simulink model "path_following_control"  (R2021a)
settings: Solver=VariableStepAuto  StartTime=0.0  StopTime=sim_time  RelTol=1e-3
values from neighbouring files (symbols this model uses):
  amax_ego = 3    [Combined_Control_Model.m]
  amin_ego = -3    [Combined_Control_Model.m]
  Cf = 155494.663    [Combined_Control_Model.m]
  Cr = 1554494.663    [Combined_Control_Model.m]
  D_default = 10    [Combined_Control_Model.m]
  Iz = 1436.24    [Combined_Control_Model.m]
  lf = 1.165    [Combined_Control_Model.m]
  lr = 1.165    [Combined_Control_Model.m]
  m = 1140    [Combined_Control_Model.m]
  t_gap = 1.4    [Combined_Control_Model.m]
  Ts = 0.1    [Combined_Control_Model.m]
  u_max = 0.5    [Combined_Control_Model.m]
  u_min = -0.5    [Combined_Control_Model.m]
  v0_ego = 25    [Combined_Control_Model.m]
  v0_lead = 25    [Combined_Control_Model.m]
  v_set = 35    [Combined_Control_Model.m]
  x0_ego = 10    [Combined_Control_Model.m]
  x0_lead = 50    [Combined_Control_Model.m]
undefined symbols (not defined in the file or in its folder): md
libraries: mpclib x1
settings Model: Creator=User  LastModifiedBy=User

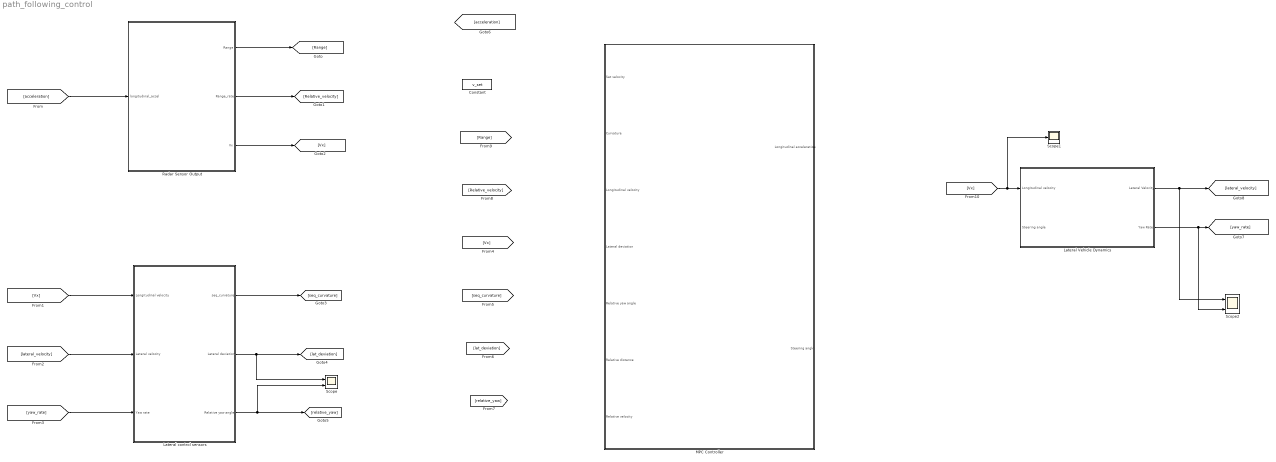
== system path_following_control ==
  Constant : Constant  Value=v_set
  Lateral Vehicle Dynamics : Subsystem
  Lateral control sensors : Subsystem
  MPC Controller : Subsystem
  Radar Sensor Output : Subsystem
  Scope : Scope  NumInputPorts=2
  Scope1 : Scope
  Scope2 : Scope  NumInputPorts=2
  wires:
  Radar Sensor Output/1(Range) -> [Range]
  Radar Sensor Output/2(Range_rate) -> [Relative_velocity]
  Radar Sensor Output/3(Vx) -> [Vx]
  Lateral control sensors/1(seq_curvature) -> [seq_curvature]
  Lateral control sensors/2(Lateral deviation) -> Scope/1, [lat_deviation]
  Lateral control sensors/3(Relative yaw angle) -> Scope/2, [relative_yaw]
  [acceleration] -> Radar Sensor Output/1(longitudinal_accel)
  [yaw_rate] -> Lateral control sensors/3(Yaw rate)
  [lateral_velocity] -> Lateral control sensors/2(Lateral velocity)
  [Vx] -> Lateral control sensors/1(Longitudinal velocity)
  [Vx] -> Lateral Vehicle Dynamics/1(Longitudinal velocity), Scope1/1
  Lateral Vehicle Dynamics/1(Lateral Velocity) -> [lateral_velocity], Scope2/1
  Lateral Vehicle Dynamics/2(Yaw Rate) -> Scope2/2, [yaw_rate]

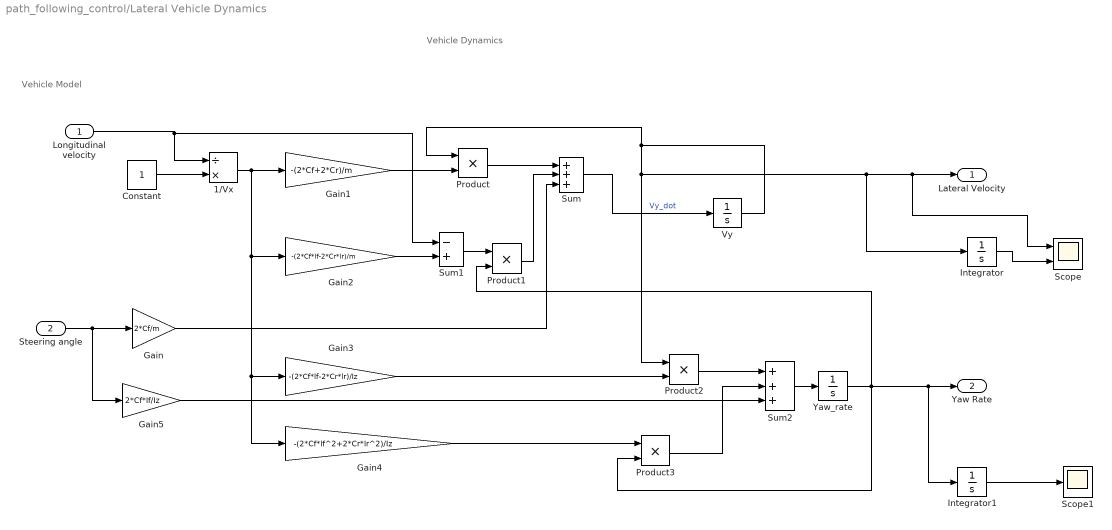
== system path_following_control/Lateral Vehicle Dynamics ==
  note: Vehicle Model
  note: Vehicle Dynamics
  Longitudinal velocity : Inport
  Steering angle : Inport  Port=2
  1/Vx : Product  Inputs=/*
  Constant : Constant
  Gain : Gain  Gain=2*Cf/m
  Gain1 : Gain  Gain=-(2*Cf+2*Cr)/m
  Gain2 : Gain  Gain=-(2*Cf*lf-2*Cr*lr)/m
  Gain3 : Gain  Gain=-(2*Cf*lf-2*Cr*lr)/Iz
  Gain4 : Gain  Gain=-(2*Cf*lf^2+2*Cr*lr^2)/Iz
  Gain5 : Gain  Gain=2*Cf*lf/Iz
  Integrator : Integrator
  Integrator1 : Integrator
  Product{,1..3} (4 alike) : Product
  Scope : Scope  NumInputPorts=2
  Scope1 : Scope
  Sum : Sum  Inputs=+++
  Sum1 : Sum  Inputs=-+
  Sum2 : Sum  Inputs=+++
  Vy : Integrator
  "Yaw_rate " : Integrator
  Lateral Velocity : Outport  VectorParamsAs1DForOutWhenUnconnected=off
  Yaw Rate : Outport  Port=2  VectorParamsAs1DForOutWhenUnconnected=off
  wires:
  Sum2/1 -> "Yaw_rate "/1
  Gain2/1 -> Sum1/2
  Gain4/1 -> Product3/1
  Constant/1 -> 1/Vx/2
  Gain3/1 -> Product2/2
  1/Vx/1 -> Gain4/1, Gain3/1, Gain2/1, Gain1/1
  Product2/1 -> Sum2/1
  Product3/1 -> Sum2/2
  Gain5/1 -> Sum2/3
  Sum1/1 -> Product1/1
  "Yaw_rate "/1 -> Product3/2, Integrator1/1, Yaw Rate/1, Product1/2
  Gain/1 -> Sum/3
  Steering angle/1 -> Gain/1, Gain5/1
  Gain1/1 -> Product/2
  Product/1 -> Sum/1
  Vy/1 -> Product/1, Integrator/1, Scope/1, Lateral Velocity/1, Product2/1
  Sum/1 -> Vy/1  "Vy_dot"
  Longitudinal velocity/1 -> Sum1/1, 1/Vx/1
  Product1/1 -> Sum/2
  Integrator/1 -> Scope/2
  Integrator1/1 -> Scope1/1

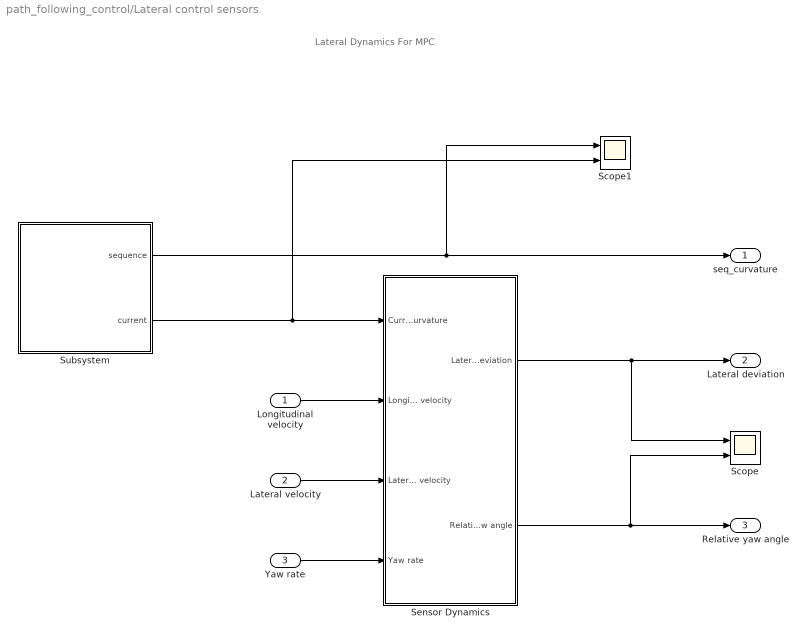
== system path_following_control/Lateral control sensors ==
  note: Lateral Dynamics For MPC
  Longitudinal velocity : Inport
  Lateral velocity : Inport  Port=2
  Yaw rate : Inport  Port=3
  Scope : Scope  NumInputPorts=2
  Scope1 : Scope  NumInputPorts=2
  Sensor Dynamics : Subsystem
  Subsystem : Subsystem  mask{signal=md, ts=Ts, steps=10}
      mask prompts: signal "Signal name"; ts "Sampling time"; steps "Number of previewing steps"
      mask init:
      | ts = evalin('base',get_param(gcbh,'ts'));
      | signal = evalin('base',get_param(gcbh,'signal'));
      | steps = evalin('base',get_param(gcbh,'steps'));
      | data = mpc_previewer_maskinit(signal,ts);
      mask Display:
      | fprintf('Future\nsample\nextractor');
      | port_label('output', 1, 'seq')
      | port_label('output', 2, '@t')
  seq_curvature : Outport
  Lateral deviation : Outport  Port=2
  Relative yaw angle : Outport  Port=3
  wires:
  Lateral velocity/1 -> Sensor Dynamics/3(Lateral velocity)
  Subsystem/2(current) -> Sensor Dynamics/1(Current curvature), Scope1/2
  Yaw rate/1 -> Sensor Dynamics/4(Yaw rate)
  Sensor Dynamics/1(Lateral deviation) -> Scope/1, Lateral deviation/1
  Sensor Dynamics/2(Relative yaw angle) -> Scope/2, Relative yaw angle/1
  Subsystem/1(sequence) -> Scope1/1, seq_curvature/1
  Longitudinal velocity/1 -> Sensor Dynamics/2(Longitudinal velocity)

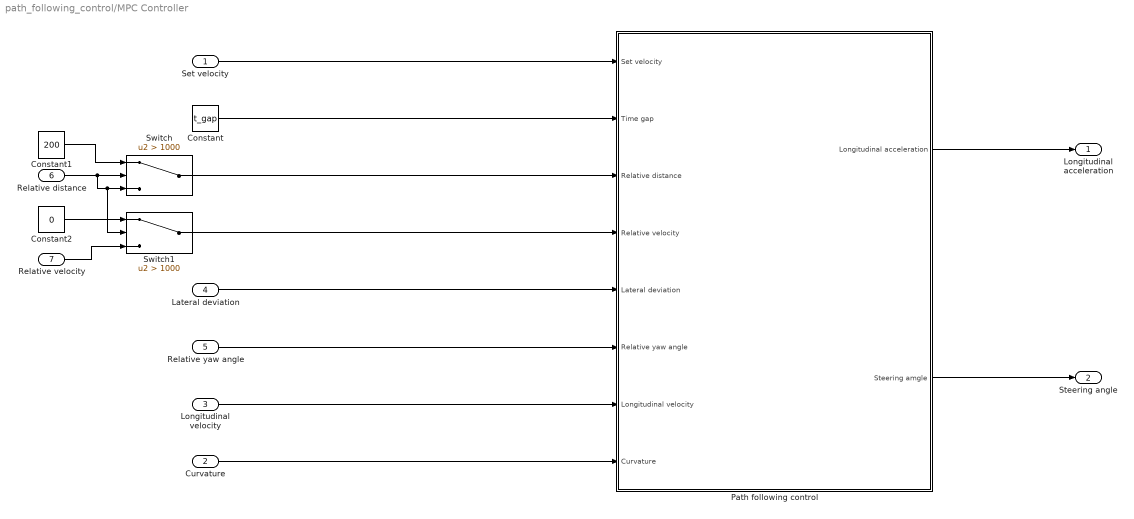
== system path_following_control/MPC Controller ==
  Set velocity : Inport
  Curvature : Inport  Port=2
  Longitudinal velocity : Inport  Port=3
  Lateral deviation : Inport  Port=4
  Relative yaw angle : Inport  Port=5
  Relative distance : Inport  Port=6
  Relative velocity : Inport  Port=7
  Constant : Constant  Value=t_gap
  Constant1 : Constant  Value=200
  Constant2 : Constant  Value=0
  Path following control : Subsystem
  Switch : Switch  Criteria=u2 > Threshold  Threshold=1000
  Switch1 : Switch  Criteria=u2 > Threshold  Threshold=1000
  Longitudinal acceleration : Outport
  Steering angle : Outport  Port=2
  wires:
  Set velocity/1 -> Path following control/1(Set velocity)
  Constant/1 -> Path following control/2(Time gap)
  Curvature/1 -> Path following control/8(Curvature)
  Longitudinal velocity/1 -> Path following control/7(Longitudinal velocity)
  Relative yaw angle/1 -> Path following control/6(Relative yaw angle)
  Lateral deviation/1 -> Path following control/5(Lateral deviation)
  Constant1/1 -> Switch/1
  Relative distance/1 -> Switch1/2, Switch/3, Switch/2
  Switch/1 -> Path following control/3(Relative distance)
  Constant2/1 -> Switch1/1
  Relative velocity/1 -> Switch1/3
  Switch1/1 -> Path following control/4(Relative velocity)
  Path following control/1(Longitudinal acceleration) -> Longitudinal acceleration/1
  Path following control/2(Steering amgle) -> Steering angle/1

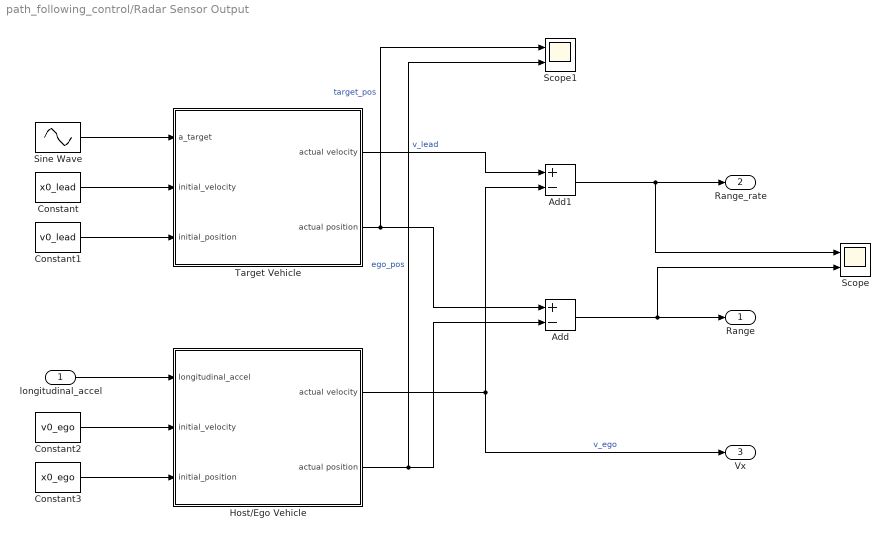
== system path_following_control/Radar Sensor Output ==
  longitudinal_accel : Inport
  Add : Sum  Inputs=+-
  Add1 : Sum  Inputs=+-
  Constant : Constant  Value=x0_lead
  Constant1 : Constant  Value=v0_lead
  Constant2 : Constant  Value=v0_ego
  Constant3 : Constant  Value=x0_ego
  Host/Ego Vehicle : Subsystem
  Scope : Scope  NumInputPorts=2
  Scope1 : Scope  NumInputPorts=2
  Sine Wave : Sin  Amplitude=0.6  Frequency=0.5  SampleTime=Ts
  Target Vehicle : Subsystem
  Range : Outport
  Range_rate : Outport  Port=2
  Vx : Outport  Port=3
  wires:
  Sine Wave/1 -> Target Vehicle/1(a_target)
  Constant1/1 -> Target Vehicle/3(initial_position)
  Constant/1 -> Target Vehicle/2(initial_velocity)
  Constant2/1 -> Host/Ego Vehicle/2(initial_velocity)
  Constant3/1 -> Host/Ego Vehicle/3(initial_position)
  longitudinal_accel/1 -> Host/Ego Vehicle/1(longitudinal_accel)
  Host/Ego Vehicle/2(actual position) -> Scope1/2, Add/2  "ego_pos"
  Target Vehicle/2(actual position) -> Scope1/1, Add/1  "target_pos"
  Add/1 -> Scope/2, Range/1
  Add1/1 -> Scope/1, Range_rate/1
  Host/Ego Vehicle/1(actual velocity) -> Vx/1, Add1/2  "v_ego"
  Target Vehicle/1(actual velocity) -> Add1/1  "v_lead"

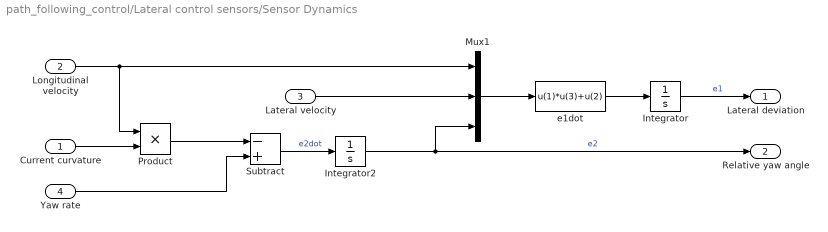
== system path_following_control/Lateral control sensors/Sensor Dynamics ==
  Current curvature : Inport
  Longitudinal velocity : Inport  Port=2
  Lateral velocity : Inport  Port=3
  Yaw rate : Inport  Port=4
  Integrator : Integrator
  Integrator2 : Integrator
  Mux1 : Mux  Inputs=[1 1 1]
  Product : Product
  Subtract : Sum  Inputs=-+
  e1dot : Fcn  Expr=u(1)*u(3)+u(2)
  Lateral deviation : Outport  VectorParamsAs1DForOutWhenUnconnected=off
  Relative yaw angle : Outport  Port=2  VectorParamsAs1DForOutWhenUnconnected=off
  wires:
  Current curvature/1 -> Product/2
  Integrator2/1 -> Mux1/3, Relative yaw angle/1  "e2"
  Mux1/1 -> e1dot/1
  e1dot/1 -> Integrator/1
  Longitudinal velocity/1 -> Product/1, Mux1/1
  Lateral velocity/1 -> Mux1/2
  Integrator/1 -> Lateral deviation/1  "e1"
  Product/1 -> Subtract/1
  Yaw rate/1 -> Subtract/2
  Subtract/1 -> Integrator2/1  "e2dot"

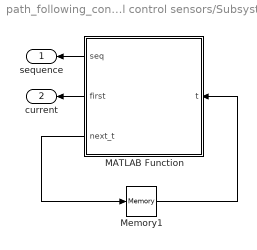
== system path_following_control/Lateral control sensors/Subsystem ==
  MATLAB Function : MATLAB Function  TreatAsAtomicUnit=on
  Memory1 : Memory  InheritSampleTime=on  LinearizeAsDelay=on
  sequence : Outport  VectorParamsAs1DForOutWhenUnconnected=off
  current : Outport  Port=2  VectorParamsAs1DForOutWhenUnconnected=off
  wires:
  MATLAB Function/2(first) -> current/1
  MATLAB Function/3(next_t) -> Memory1/1
  MATLAB Function/1(seq) -> sequence/1
  Memory1/1 -> MATLAB Function/1(t)

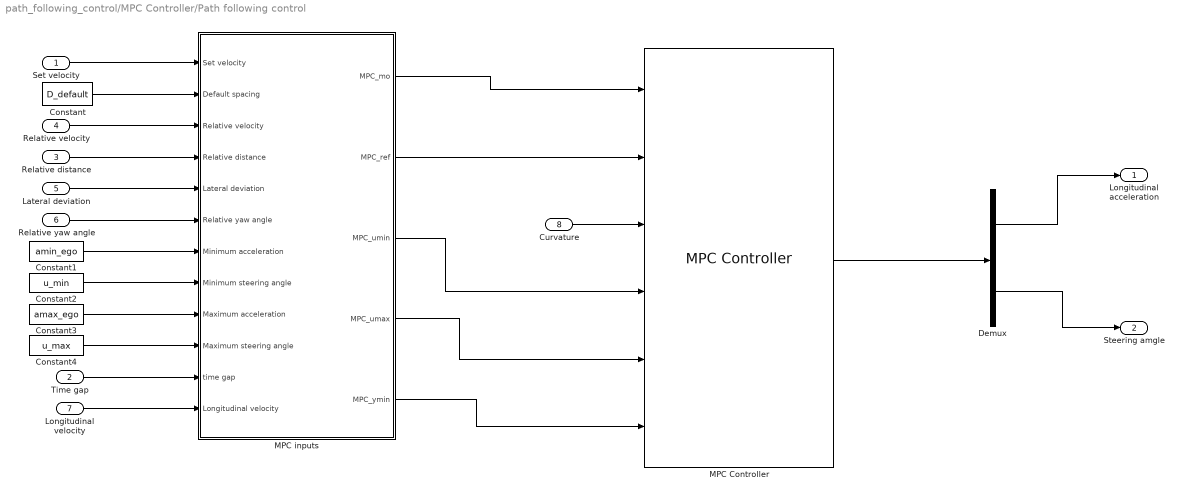
== system path_following_control/MPC Controller/Path following control ==
  Set velocity : Inport
  Time gap : Inport  Port=2
  Relative distance : Inport  Port=3
  Relative velocity : Inport  Port=4
  Lateral deviation : Inport  Port=5
  Relative yaw angle : Inport  Port=6
  Longitudinal velocity : Inport  Port=7
  Curvature : Inport  Port=8
  Constant : Constant  Value=D_default
  Constant1 : Constant  Value=amin_ego
  Constant2 : Constant  Value=u_min
  Constant3 : Constant  Value=amax_ego
  Constant4 : Constant  Value=u_max
  Demux : Demux  Outputs=2
  MPC Controller : mpclib/MPC Controller  SCDEnableBlockLinearizationSpecification=on  mpcobj=mpc1  is_multiple=0  enable_value=0  return_u0=off  updateMPCinCallerWorkspace=on  md_inport=on  mv_inport=off  uref_inport=off  return_cost=off  return_mvseq=off  return_qpstatus=off  return_xseq=off  return_state=off  return_ovseq=off  state_inport=off  umin_inport=on  umax_inport=on  ymin_inport=on  ymax_inport=off  cc_inport=off  ywt_inport=off  uwt_inport=off  duwt_inport=off  rhoeps_inport=off  pm_inport=off  MaximumP=10  HorizonChoice=FixedHorizon  n_ts=1  n_p=10  n_mv=1  n_md=1  n_ud=0  n_mo=1  n_uo=0  BlockDataType=double  SampleTimeInherited=off  switch_inport=off
  MPC inputs : Subsystem
  Longitudinal acceleration : Outport
  Steering amgle : Outport  Port=2
  wires:
  MPC inputs/1(MPC_mo) -> MPC Controller/1
  MPC inputs/2(MPC_ref) -> MPC Controller/2
  MPC inputs/3(MPC_umin) -> MPC Controller/4
  MPC inputs/4(MPC_umax) -> MPC Controller/5
  MPC inputs/5(MPC_ymin) -> MPC Controller/6
  MPC Controller/1 -> Demux/1
  Demux/1 -> Longitudinal acceleration/1
  Demux/2 -> Steering amgle/1
  Set velocity/1 -> MPC inputs/1(Set velocity)
  Curvature/1 -> MPC Controller/3
  Constant/1 -> MPC inputs/2(Default spacing)
  Relative velocity/1 -> MPC inputs/3(Relative velocity)
  Time gap/1 -> MPC inputs/11(time gap)
  Relative distance/1 -> MPC inputs/4(Relative distance)
  Lateral deviation/1 -> MPC inputs/5(Lateral deviation)
  Relative yaw angle/1 -> MPC inputs/6(Relative yaw angle)
  Longitudinal velocity/1 -> MPC inputs/12(Longitudinal velocity)
  Constant1/1 -> MPC inputs/7(Minimum acceleration)
  Constant2/1 -> MPC inputs/8(Minimum steering angle)
  Constant3/1 -> MPC inputs/9(Maximum acceleration)
  Constant4/1 -> MPC inputs/10(Maximum steering angle)

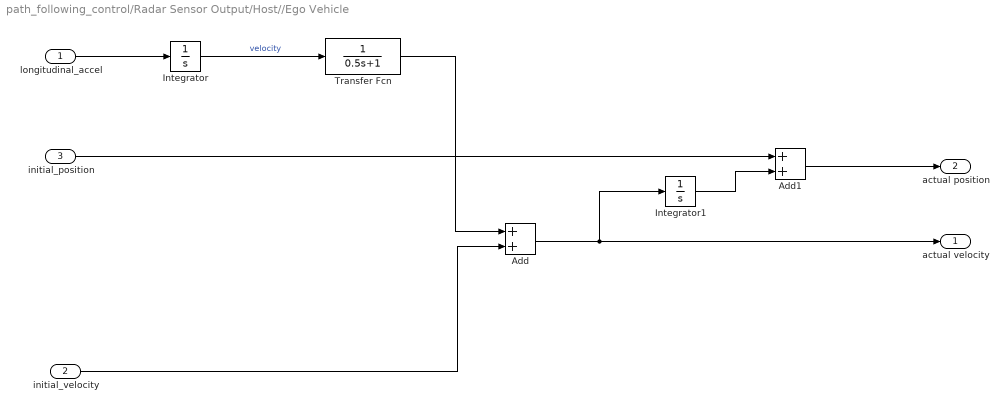
== system path_following_control/Radar Sensor Output/Host//Ego Vehicle ==
  longitudinal_accel : Inport
  initial_velocity : Inport  Port=2
  initial_position : Inport  Port=3
  Add : Sum
  Add1 : Sum
  Integrator : Integrator
  Integrator1 : Integrator
  Transfer Fcn : TransferFcn  Denominator=[0.5 1]
  actual velocity : Outport
  actual position : Outport  Port=2
  wires:
  Add1/1 -> actual position/1
  initial_position/1 -> Add1/1
  Integrator1/1 -> Add1/2
  Add/1 -> actual velocity/1, Integrator1/1
  initial_velocity/1 -> Add/2
  Transfer Fcn/1 -> Add/1
  Integrator/1 -> Transfer Fcn/1  "velocity"
  longitudinal_accel/1 -> Integrator/1

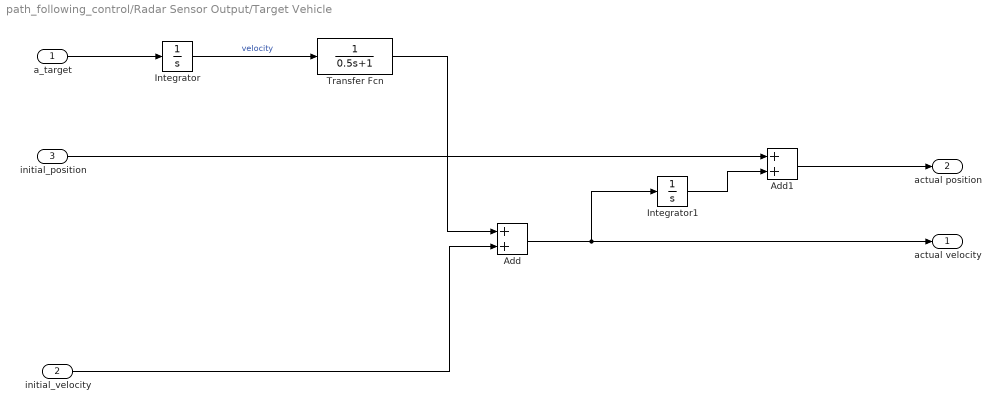
== system path_following_control/Radar Sensor Output/Target Vehicle ==
  a_target : Inport
  initial_velocity : Inport  Port=2
  initial_position : Inport  Port=3
  Add : Sum
  Add1 : Sum
  Integrator : Integrator
  Integrator1 : Integrator
  Transfer Fcn : TransferFcn  Denominator=[0.5 1]
  actual velocity : Outport
  actual position : Outport  Port=2
  wires:
  a_target/1 -> Integrator/1
  Integrator/1 -> Transfer Fcn/1  "velocity"
  Transfer Fcn/1 -> Add/1
  initial_velocity/1 -> Add/2
  Add/1 -> Integrator1/1, actual velocity/1
  Integrator1/1 -> Add1/2
  initial_position/1 -> Add1/1
  Add1/1 -> actual position/1

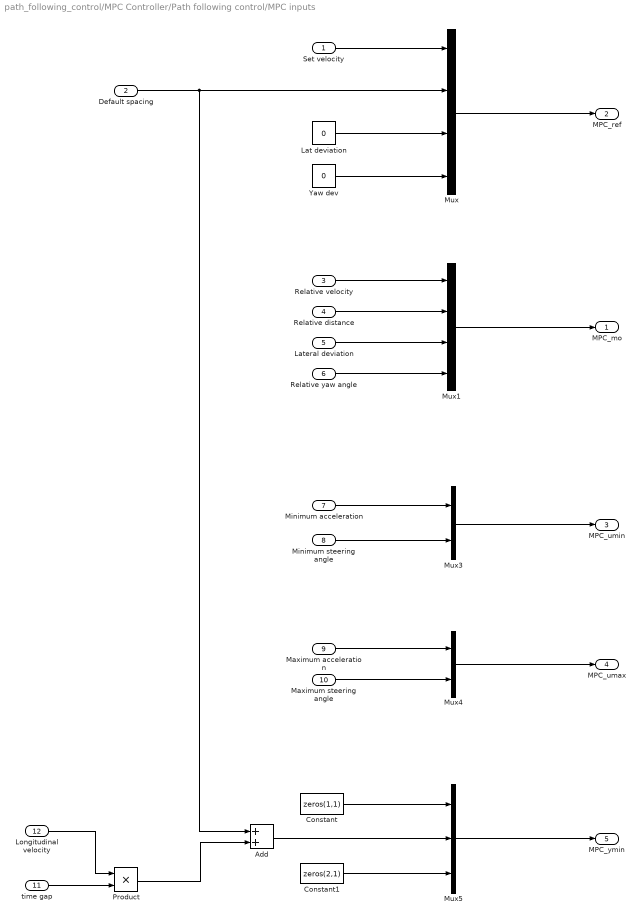
== system path_following_control/MPC Controller/Path following control/MPC inputs ==
  Set velocity : Inport
  Default spacing : Inport  Port=2
  Relative velocity : Inport  Port=3
  Relative distance : Inport  Port=4
  Lateral deviation : Inport  Port=5
  Relative yaw angle : Inport  Port=6
  Minimum acceleration : Inport  Port=7
  Minimum steering angle : Inport  Port=8
  Maximum acceleration : Inport  Port=9
  Maximum steering angle : Inport  Port=10
  time gap : Inport  Port=11
  Longitudinal velocity : Inport  Port=12
  Add : Sum
  Constant : Constant  Value=zeros(1,1)
  Constant1 : Constant  Value=zeros(2,1)
  Lat deviation : Constant  Value=0
  Mux : Mux
  Mux1 : Mux
  Mux3 : Mux  Inputs=2
  Mux4 : Mux  Inputs=2
  Mux5 : Mux  Inputs=3
  Product : Product
  Yaw dev : Constant  Value=0
  MPC_mo : Outport
  MPC_ref : Outport  Port=2
  MPC_umin : Outport  Port=3
  MPC_umax : Outport  Port=4
  MPC_ymin : Outport  Port=5
  wires:
  Mux/1 -> MPC_ref/1
  Set velocity/1 -> Mux/1
  Default spacing/1 -> Mux/2, Add/1
  Lat deviation/1 -> Mux/3
  Yaw dev/1 -> Mux/4
  Relative velocity/1 -> Mux1/1
  Relative distance/1 -> Mux1/2
  Lateral deviation/1 -> Mux1/3
  Relative yaw angle/1 -> Mux1/4
  Mux1/1 -> MPC_mo/1
  Mux3/1 -> MPC_umin/1
  Minimum acceleration/1 -> Mux3/1
  Minimum steering angle/1 -> Mux3/2
  Maximum acceleration/1 -> Mux4/1
  Maximum steering angle/1 -> Mux4/2
  Mux4/1 -> MPC_umax/1
  Mux5/1 -> MPC_ymin/1
  Constant/1 -> Mux5/1
  Constant1/1 -> Mux5/3
  time gap/1 -> Product/2
  Longitudinal velocity/1 -> Product/1
  Product/1 -> Add/2
  Add/1 -> Mux5/2

== matlab function path_following_control/Lateral control sensors/Subsystem/MATLAB Function ==
  settings: updateMethod=DISCRETE  sampleTime=ts
  data: data parameter; seq output; steps parameter; t input; first output; next_t output
function [seq,first,next_t] = fcn(data,steps,t)
%#codegen
[seq,first,next_t] = mpcblock_preview('md',data,steps,t);
